simulink model "RLS"  (R2024a)
settings: Solver=FixedStepAuto  StartTime=0.0  StopTime=100  FixedStep=0.001  RelTol=1e-3
libraries: ctrlSharedLib x1
settings Model: Creator=rocke  LastModifiedBy=rocke

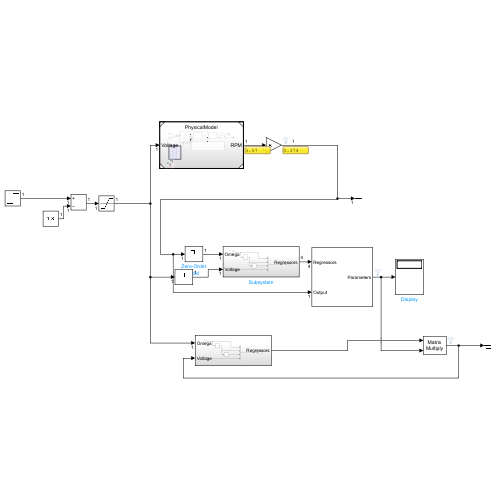
[thumbnail: Simulink's stored preview of the top-level diagram]
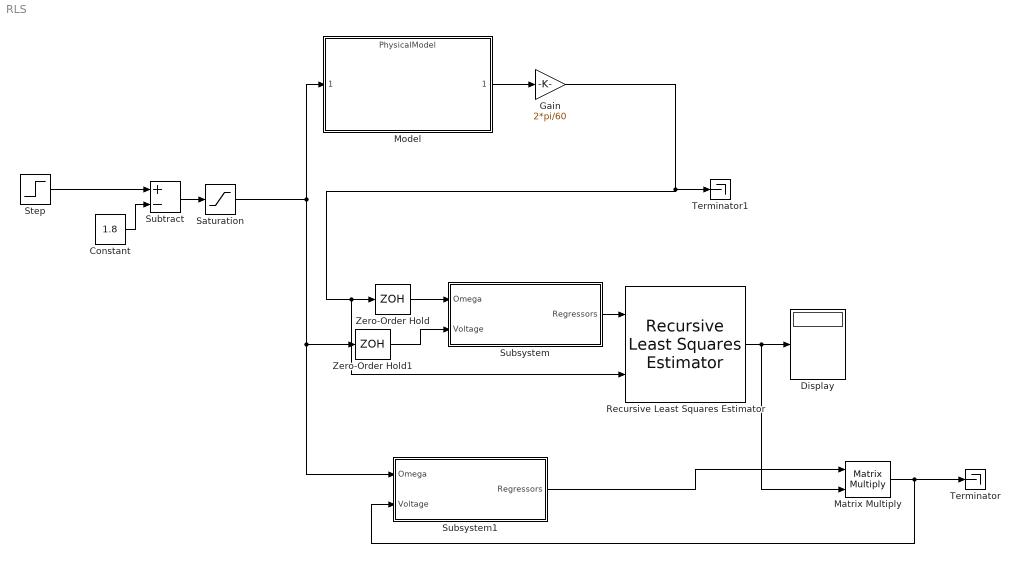
== system RLS ==
  Constant : Constant  Value=1.8
  Display : Display
  Gain : Gain  Gain=2*pi/60
  Matrix Multiply : Product  Multiplication=Matrix(*)
  Model : ModelReference  ModelNameDialog=PhysicalModel.slx  SimulationMode=Normal  ModelReferenceVersion=1.23
  Recursive Least Squares Estimator : ctrlSharedLib/Recursive Least Squares Estimator  InitialEstimateSource=None  InitialParameterData=3  P0=1e4  InitialRegressors=0  InitialOutputs=0  History=Infinite  WindowLength=200  EstimationMethod=Kalman Filter  AdaptationParameter=1  HasTimeVaryingAdaptationParameter=off  NormalizationBias=eps  OutputError=off  OutputP=off  AddEnablePort=off  InputProcessing=Sample-based  Ts=-1
      settings: LibrarySourceBlock=slident/Estimators/Recursive Least Squares Estimator
  Saturation : Saturate  UpperLimit=inf  LowerLimit=0
  Step : Step  After=12  SampleTime=0
  Subsystem : Subsystem
  Subsystem1 : Subsystem
  Subtract : Sum  Inputs=+-
  Terminator : Terminator
  Terminator1 : Terminator
  Zero-Order Hold : ZeroOrderHold  SampleTime=-1
  Zero-Order Hold1 : ZeroOrderHold  SampleTime=-1
  wires:
  Model/1 -> Gain/1
  Saturation/1 -> Subsystem1/1(Omega), Zero-Order Hold1/1, Model/1
  Step/1 -> Subtract/1
  Subtract/1 -> Saturation/1
  Constant/1 -> Subtract/2
  Subsystem/1(Regressors) -> Recursive Least Squares Estimator/1
  Gain/1 -> Recursive Least Squares Estimator/2, Zero-Order Hold/1, Terminator1/1
  Recursive Least Squares Estimator/1 -> Matrix Multiply/2, Display/1
  Matrix Multiply/1 -> Subsystem1/2(Voltage), Terminator/1
  Zero-Order Hold/1 -> Subsystem/1(Omega)
  Zero-Order Hold1/1 -> Subsystem/2(Voltage)
  Subsystem1/1(Regressors) -> Matrix Multiply/1

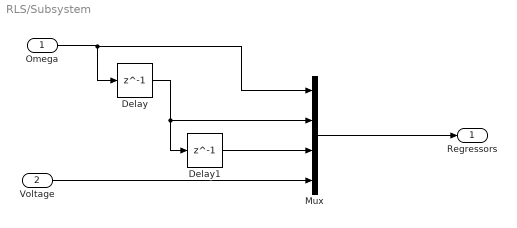
== system RLS/Subsystem ==
  Omega : Inport
  Voltage : Inport  Port=2
  Delay : Delay  DelayLength=1
  Delay1 : Delay  DelayLength=1
  Mux : Mux
  Regressors : Outport
  wires:
  Delay/1 -> Mux/2, Delay1/1
  Omega/1 -> Mux/1, Delay/1
  Mux/1 -> Regressors/1
  Voltage/1 -> Mux/4
  Delay1/1 -> Mux/3

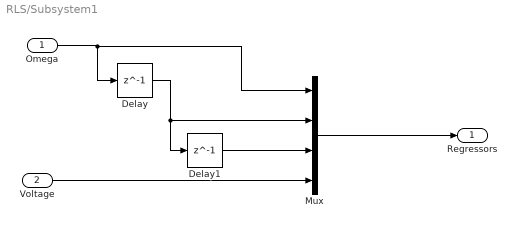
== system RLS/Subsystem1 ==
  Omega : Inport
  Voltage : Inport  Port=2
  Delay : Delay  DelayLength=1
  Delay1 : Delay  DelayLength=1
  Mux : Mux
  Regressors : Outport
  wires:
  Voltage/1 -> Mux/4
  Mux/1 -> Regressors/1
  Delay/1 -> Mux/2, Delay1/1
  Omega/1 -> Mux/1, Delay/1
  Delay1/1 -> Mux/3
